simulink model "Copy_of_NDI"  (R2024b)
settings: Solver=ode4  StartTime=0  StopTime=100  FixedStep=fcs.Ts  RelTol=1e-3
PreLoadFcn:
  | FlightPhase = 'FallingLeaf';
  | % FlightPhase = 'InAir';
  | % FlightPhase = 'TVC_h10000V617alpha2';
  | run('PreLoadFcn.m')
values from neighbouring files (symbols this model uses):
  ControlAllocation = 1    [PreLoadFcn.m]    (also in RunThis_ChiaWei.m = 4; RunThis_LM.m = 4; RunThis_Shao.m; RunThis_james.m = 10)
  DUmax = IN_MAT(k+4,1:m)'    [LP_def.m]    (also in LP_lift.m; LP_sig.m; LP_thrust.m; PreLoadFcn.m = [Aactuator.right_aileron.RateLimitUpper Aactuator.left_ailer)
  DUmin = IN_MAT(k+5,1:m)'    [LP_def.m]    (also in LP_lift.m; LP_sig.m; LP_thrust.m; PreLoadFcn.m = [Aactuator.right_aileron.RateLimitLower Aactuator.left_ailer)
  g = [ 0  0  32.17 ]    [PreLoadFcn.m]
  hground = 0    [PreLoadFcn.m]
  m = m1-1    [CGIwrap.m]    (also in DAISY_CHAINING.m; DA_Allocation.m; LP_BasicSolution.m; LP_def.m)
  Mode_deflection_aileron = 1    [PreLoadFcn.m]    (also in RunThis_ChiaWei.m; RunThis_Shao.m = 0)
  Mode_deflection_elevator = 1    [PreLoadFcn.m]    (also in RunThis_ChiaWei.m; RunThis_Shao.m = 0)
  Mode_deflection_rudder = 1    [PreLoadFcn.m]    (also in RunThis_ChiaWei.m; RunThis_Shao.m = 0)
  Mode_deflection_TVC_y = 1    [PreLoadFcn.m]    (also in RunThis_ChiaWei.m; RunThis_Shao.m = 2)
  Mode_deflection_TVC_z = 1    [PreLoadFcn.m]    (also in RunThis_ChiaWei.m; RunThis_Shao.m = 0)
  N = IN_MAT(k+7:k+15,1:m)    [CGIwrap.m]    (also in DAISY_CHAINING.m; PreLoadFcn.m = [ 1      0     0.25; RunThis_ChiaWei.m = [ 1      0     0.25; RunThis_LM.m = [ 1      0     0.25)
  Ninv_2nozzle = inv(diag([  1/21.5  1/21.5  1/25  1/25  1/30  1/15  1/15  1/15  1/15 ]))    [PreLoadFcn.m]
  Ninv_no_nozzle = diag([    21.5    21.5    25    25    30    0     0     0     0  ])    [PreLoadFcn.m]
  state0 = [IC.npos IC.epos IC.alt IC.q0 IC.q1 IC.q2 IC.q3  IC.p IC.q IC.r IC.alpha IC.beta IC.mu IC.Vt IC.chi IC.gamma]    [PreLoadFcn.m]
  Umax_2nozzle = [Aactuator.right_aileron.AngleLimitUpper  Aactuator.left_aileron.AngleLimitUpper  Aactuator.right_elevator.AngleLimitUpper Aactuator.left_elevator.AngleLimitUpper  Aactuator.rudder.AngleLimitUpper                  Aactuator.TVC_ry.AngleLimitUpper    Aactuator.TVC_rz.AngleLimitUpper  Aactuator.TVC_ly.AngleLimitUpper    Aactuator.TVC_lz.AngleLimitUpper]    [PreLoadFcn.m]
  Umax_no_nozzle = [Aactuator.right_aileron.AngleLimitUpper  Aactuator.left_aileron.AngleLimitUpper  Aactuator.right_elevator.AngleLimitUpper Aactuator.left_elevator.AngleLimitUpper  Aactuator.rudder.AngleLimitUpper                    0 0 0 0]    [PreLoadFcn.m]
  Umin_2nozzle = [Aactuator.aileron.AngleLimitLower  Aactuator.aileron.AngleLimitLower  Aactuator.elevator.AngleLimitLower Aactuator.elevator.AngleLimitLower  Aactuator.rudder.AngleLimitLower                  Aactuator.TVC_ry.AngleLimitLower    Aactuator.TVC_rz.AngleLimitLower Aactuator.TVC_ly.AngleLimitLower    Aactuator.TVC_lz.AngleLimitLower]    [PreLoadFcn.m]
  Umin_no_nozzle = [Aactuator.right_aileron.AngleLimitLower  Aactuator.left_aileron.AngleLimitLower  Aactuator.right_elevator.AngleLimitLower Aactuator.left_elevator.AngleLimitLower  Aactuator.rudder.AngleLimitLower                    0 0 0 0]    [PreLoadFcn.m]
undefined symbols (not defined in the file or in its folder): Aactuator, ac, AeroCoeff, EngineTable, F, fcs, ft, IC, kg, LandingGear, Light, MIL, PIController, s, Sensor, sigbuilder_block, slug, sysID_DAQ, sysID_OBES, WMM2020
libraries: aerolibconvert2 x31, slpidlib x11, simulink x6, sharedutil x4, aerolibatmos2 x3, aerolibwind2 x3, aerolibbdyn x3, aerolibgravity2 x2, sharedtransform x1
(part 13 of 14)

== system Copy_of_NDI/F-16 Vehicle Systems Model/Vehicle/Aerodynamics/Aerofynamic Coefficients/CZT ==
  note: 氣動力表格僅提供到攻角到
      | 45度，超過45度後皆採用45
      | 度的氣動力係數
  note: ${\hat{Z} }_{\delta_e } =\frac{C_Z {\left(\alpha ,\beta ,\delta_e +0.1\right)}-C_Z {\left(\alpha ,\beta ,\delta_e -0.1\right)}}{0.2}$
  note: $\Delta C_{Z_{LEF} } =C_{Z_{LEF} } {\left(\alpha ,\beta \right)}-C_Z {\left(\alpha ,\beta ,\delta_e =0°\right)}$
  note: $C_{Z,T} =C_Z {\left(\alpha ,\beta ,\delta_e \right)}+\Delta C_{Z_{LEF} } ∙{\left(1-\frac{\delta_{LEF} }{25°}\right)}+\frac{q\overset{-}{c} }{2V_T }∙{\left[C_{Z_q } {\left(\alpha \right)}+\Delta C_{Z_{q_{LEF} } } {\left(\alpha \right)}∙{\left(1-\frac{\delta_{LEF} }{25°}\right)}\right]}+\ \Delta C_{Z_{SB} } {\left(\alpha \right)}∙{\left(\frac{\delta_{SB} }{60°}\right)}+C_{Z_{\delta ra} } \delta_{ra} +C_{Z_{\delta la} } \delta_{la}$
  note: $C_{Z_{\delta ra} } =C_{Z_{\delta la} } =\frac{{\hat{Z} }_{\delta_e } }{2}∙0.4$
  note: 體軸 z 方向之氣動力係數 (total z-axis force coefficient)：
  note: ${\hat{Z} }_{\delta_e } =\frac{C_Z {\left(\alpha ,\beta ,\delta_e +0.1\right)}-C_Z {\left(\alpha ,\beta ,\delta_e -0.1\right)}}{0.2}$
  note: $C_{Z_{\delta ra} } =C_{Z_{\delta la} } =\frac{{\hat{Z} }_{\delta_e } }{2}∙0.4$
  alpha (deg) : Inport
  beta (deg) : Inport  Port=2
  right elevator (deg) : Inport  Port=3
  left elevator (deg) : Inport  Port=4
  dlef : Inport  Port=5
  qc_2v : Inport  Port=6
  sb : Inport  Port=7
  right aileron : Inport  Port=8
  left aileron : Inport  Port=9
  Add : Sum  Inputs=+-
  Add1 : Sum  Inputs=+++++
  Add{2..4,7} (4 alike) : Sum
  Add5 : Sum  Inputs=+-
  Add6 : Sum  Inputs=+-
  CZ : Interpolation_n-D  NumberOfTableDimensions=3  Table=AeroCoeff.CZ
      settings: InputPortMap=u0,u1,u2,u3,u4,u5
  CZ1 : Interpolation_n-D  NumberOfTableDimensions=3  Table=AeroCoeff.CZ
      settings: InputPortMap=u0,u1,u2,u3,u4,u5
  CZ2 : Interpolation_n-D  NumberOfTableDimensions=3  Table=AeroCoeff.CZ
      settings: InputPortMap=u0,u1,u2,u3,u4,u5
  CZ_elevator0 : Interpolation_n-D  Table=AeroCoeff.CZ_elevator0
  CZ_lef : Interpolation_n-D  Table=AeroCoeff.CZ_lef
  CZ_q : Interpolation_n-D  NumberOfTableDimensions=1  Table=AeroCoeff.CZ_q
      settings: InputPortMap=u0,u1
  Constant : Constant  Value=0.1
  Constant1 : Constant  Value=0.1
  Constant2 : Constant  Value=0.2
  Divide : Product  Inputs=*/
  Gain : Gain  Gain=20
  Gain2 : Gain  Gain=(1/2)*0.4
  Gain3 : Gain  Gain=20
  Gain4 : Gain  Gain=1/2
  Product{,1..5} (6 alike) : Product
  alpha Prelookup : PreLookup  BreakpointsData=AeroCoeff.alpha_prelookup  IndexSearchMethod=Linear search  BeginIndexSearchUsingPreviousIndexResult=on  DiagnosticForOutOfRangeInput=Warning
  beta Prelookup : PreLookup  BreakpointsData=AeroCoeff.beta_prelookup  IndexSearchMethod=Linear search  BeginIndexSearchUsingPreviousIndexResult=on  DiagnosticForOutOfRangeInput=Warning
  dCZ_q_lef : Interpolation_n-D  NumberOfTableDimensions=1  Table=AeroCoeff.dCZ_q_lef
      settings: InputPortMap=u0,u1
  dCZ_sb : Interpolation_n-D  NumberOfTableDimensions=1  Table=AeroCoeff.dCZ_sb
      settings: InputPortMap=u0,u1
  elevator Prelookup : PreLookup  BreakpointsData=AeroCoeff.elevator_prelookup2  IndexSearchMethod=Linear search  BeginIndexSearchUsingPreviousIndexResult=on  DiagnosticForOutOfRangeInput=Warning
  elevator Prelookup1 : PreLookup  BreakpointsData=AeroCoeff.elevator_prelookup2  IndexSearchMethod=Linear search  BeginIndexSearchUsingPreviousIndexResult=on  DiagnosticForOutOfRangeInput=Warning
  elevator Prelookup2 : PreLookup  BreakpointsData=AeroCoeff.elevator_prelookup2  IndexSearchMethod=Linear search  BeginIndexSearchUsingPreviousIndexResult=on  DiagnosticForOutOfRangeInput=Warning
  Cz_tot : Outport  VectorParamsAs1DForOutWhenUnconnected=off
  wires:
  Product2/1 -> Add1/3
  alpha Prelookup/2 -> dCZ_q_lef/2, dCZ_sb/2, CZ2/2, CZ1/2, CZ_q/2, CZ_elevator0/2, CZ_lef/2, CZ/2
  Add1/1 -> Cz_tot/1
  elevator Prelookup/1 -> CZ/5
  CZ_q/1 -> Add2/1
  beta Prelookup/2 -> CZ/4, CZ_lef/4, CZ_elevator0/4, CZ2/4, CZ1/4
  CZ_lef/1 -> Add/1
  dCZ_q_lef/1 -> Product1/1
  Product1/1 -> Add2/2
  Add2/1 -> Product2/1
  CZ_elevator0/1 -> Add/2
  Add/1 -> Product/1
  dlef/1 -> Product1/2, Product/2
  Product/1 -> Add1/2
  CZ/1 -> Add1/1
  beta Prelookup/1 -> CZ/3, CZ_elevator0/3, CZ2/3, CZ1/3, CZ_lef/3
  alpha Prelookup/1 -> dCZ_q_lef/1, CZ1/1, CZ2/1, dCZ_sb/1, CZ_q/1, CZ_elevator0/1, CZ_lef/1, CZ/1
  alpha (deg)/1 -> alpha Prelookup/1
  elevator Prelookup/2 -> CZ/6
  qc_2v/1 -> Product2/2
  beta (deg)/1 -> beta Prelookup/1
  sb/1 -> Product3/2
  dCZ_sb/1 -> Product3/1
  Product3/1 -> Add1/4
  Constant1/1 -> Add5/2
  CZ2/1 -> Add6/2
  Constant/1 -> Add4/2
  Add5/1 -> elevator Prelookup2/1
  Product5/1 -> Add7/2
  Add4/1 -> elevator Prelookup1/1
  left aileron/1 -> Gain3/1
  Divide/1 -> Gain2/1
  right aileron/1 -> Gain/1
  Add6/1 -> Divide/1
  Gain2/1 -> Product5/1, Product4/1
  CZ1/1 -> Add6/1
  Product4/1 -> Add7/1
  Add3/1 -> Gain4/1
  right elevator (deg)/1 -> Add3/1
  left elevator (deg)/1 -> Add3/2
  elevator Prelookup1/1 -> CZ1/5
  elevator Prelookup1/2 -> CZ1/6
  elevator Prelookup2/1 -> CZ2/5
  elevator Prelookup2/2 -> CZ2/6
  Constant2/1 -> Divide/2
  Add7/1 -> Add1/5
  Gain/1 -> Product4/2
  Gain3/1 -> Product5/2
  Gain4/1 -> elevator Prelookup/1, Add5/1, Add4/1

== system Copy_of_NDI/F-16 Vehicle Systems Model/Vehicle/Aerodynamics/Aerofynamic Coefficients/ClT ==
  note: $\Delta C_{l_{\delta_a } }$
  note: $\Delta C_{l_{{\delta_a }_{LEF} } } =C_{l_{{\delta_a =20°}_{LEF} } } {\left(\alpha ,\beta \right)}-C_{l_{LEF} } {\left(\alpha ,\beta \right)}-\Delta C_{l_{\delta_a } }$
  note: $\Delta C_{l_{\delta_r } } =C_{l_{\delta_r =30°} } {\left(\alpha ,\beta \right)}-C_l {\left(\alpha ,\beta ,\delta_e =0°\right)}$
  note: $\Delta C_{l_{\delta_a } } =C_{l_{\delta_a =20°} } {\left(\alpha ,\beta \right)}-C_l {\left(\alpha ,\beta ,\delta_e =0°\right)}$
  note: $\Delta C_{l_{LEF} } =C_{l_{LEF} } {\left(\alpha ,\beta \right)}-C_l {\left(\alpha ,\beta ,\delta_e =0°\right)}$
  note: 側滾氣動力矩係數 (total rolling moment coefficient)：
  note: 氣動力表格僅提供到攻角到
      | 45度，超過45度後皆採用45
      | 度的氣動力係數
  note: 氣動力表格僅提供到攻角到
      | 45度，超過45度後皆採用45
      | 度的氣動力係數
  note: $C_{l,T} \ \ \ =\ \ \ C_l {\left(\alpha ,\beta ,\delta_e \right)}+\Delta C_{l_{LEF} } ∙{\left(1-\frac{\delta_{LEF} }{25°}\right)}+\frac{pb}{2V_T }∙{\left[C_{l_p } {\left(\alpha \right)}+\Delta C_{l_{p_{LEF} } } {\left(\alpha \right)}∙{\left(1-\frac{\delta_{LEF} }{25°}\right)}\right]}+\frac{rb}{2V_T }∙{\left[C_{l_r } {\left(\alpha \right)}+\Delta C_{l_{r_{LEF} } } {\left(\alpha \right)}∙{\left(1-\frac{\delta_{LEF} }{25°}\right)}\right]}+\Delta C_{l_{\beta } } {\left(\alpha \right)}∙\beta +\Delta C_{l_{\delta_r } } ∙{\left(\frac{\delta_r }{30°}\right)}+\frac{{\left[\Delta C_{l_{\delta_a } } +\Delta C_{l_{{\delta_a }_{LEF} } } ∙{\left(1-\frac{\delta_{LEF} }{25°}\right)}\right]}}{2}∙{\left(\frac{\delta_{ra} }{20°}\right)}-\frac{{\left[\Delta C_{l_{\delta_a } } +\Delta C_{l_{{\delta_a }_{LEF} } } ∙{\left(1-\frac{\delta_{LEF} }{25°}\right)}\right]}}{2}∙{\left(\frac{\delta_{la} }{20°}\right)}+C_{l_{\delta re} } ∙{\left(\frac{\delta_{re} }{25°}\right)}-C_{l_{\delta le} } ∙{\left(\frac{\delta_{le} }{25°}\right)}$
  note: $C_{l_{\delta re} } =C_{l_{\delta le} } =\frac{\Delta C_{l_{\delta_a } } }{2}∙0.56$
  note: $\Delta C_{l_{\delta_a } }$
  note: $C_{l_{\delta re} } =C_{l_{\delta le} } =\frac{\Delta C_{l_{\delta_a } } }{2}∙0.56$
  alpha (deg) : Inport
  beta (deg) : Inport  Port=2
  drud : Inport  Port=3
  dlef : Inport  Port=4
  right aileron : Inport  Port=5
  left aileron : Inport  Port=6
  rb_2v : Inport  Port=7
  pb_2v : Inport  Port=8
  right elevator (deg) : Inport  Port=9
  left elevator (deg) : Inport  Port=10
  Add : Sum  Inputs=+-
  Add1 : Sum  Inputs=+-
  Angle Conversion : aerolibconvert2/Angle Conversion  IU=deg  OU=rad
  Cl : Interpolation_n-D  NumberOfTableDimensions=3  Table=AeroCoeff.Cl
      settings: InputPortMap=u0,u1,u2,u3,u4,u5
  Cl_delta_ail : Interpolation_n-D  Table=AeroCoeff.Cl_delta_ail  InternalRulePriority=Speed
  Cl_delta_ail_lef : Interpolation_n-D  Table=AeroCoeff.Cl_delta_ail_lef  InternalRulePriority=Speed
  Cl_delta_r : Interpolation_n-D  Table=AeroCoeff.Cl_delta_r  InternalRulePriority=Speed
  Cl_elevator0 : Interpolation_n-D  Table=AeroCoeff.Cl_elevator0
  Cl_lef : Interpolation_n-D  Table=AeroCoeff.Cl_lef  InternalRulePriority=Speed
  Cl_p : Interpolation_n-D  NumberOfTableDimensions=1  Table=AeroCoeff.Cl_p  InternalRulePriority=Speed
      settings: InputPortMap=u0,u1
  Cl_r : Interpolation_n-D  NumberOfTableDimensions=1  Table=AeroCoeff.Cl_r  InternalRulePriority=Speed
      settings: InputPortMap=u0,u1
  Gain : Gain  Gain=1/2
  Gain1 : Gain  Gain=1/25
  Gain2 : Gain  Gain=(1/2)*0.56
  Product{,1..9} (10 alike) : Product
  Subtract : Sum  Inputs=+-
  Subtract1 : Sum  Inputs=+-
  Subtract2 : Sum  Inputs=+--
  Subtract3 : Sum  Inputs=+-
  Subtract4 : Sum  Inputs=++++++++
  Subtract5 : Sum
  Subtract6 : Sum
  Subtract7 : Sum
  alpha Prelookup : PreLookup  BreakpointsData=AeroCoeff.alpha_prelookup  IndexSearchMethod=Linear search  BeginIndexSearchUsingPreviousIndexResult=on  DiagnosticForOutOfRangeInput=Warning
  beta Prelookup : PreLookup  BreakpointsData=AeroCoeff.beta_prelookup  IndexSearchMethod=Linear search  BeginIndexSearchUsingPreviousIndexResult=on  DiagnosticForOutOfRangeInput=Warning
  dCl_beta : Interpolation_n-D  NumberOfTableDimensions=1  Table=AeroCoeff.dCl_beta  InternalRulePriority=Speed
      settings: InputPortMap=u0,u1
  dCl_p_lef : Interpolation_n-D  NumberOfTableDimensions=1  Table=AeroCoeff.dCl_p_lef  InternalRulePriority=Speed
      settings: InputPortMap=u0,u1
  dCl_r_lef : Interpolation_n-D  NumberOfTableDimensions=1  Table=AeroCoeff.dCl_r_lef  InternalRulePriority=Speed
      settings: InputPortMap=u0,u1
  elevator Prelookup : PreLookup  BreakpointsData=AeroCoeff.elevator_prelookup1  IndexSearchMethod=Linear search  BeginIndexSearchUsingPreviousIndexResult=on  DiagnosticForOutOfRangeInput=Warning
  Cl_tot : Outport  VectorParamsAs1DForOutWhenUnconnected=off
  wires:
  Cl_elevator0/1 -> Subtract3/2, Subtract1/2, Subtract/2
  beta Prelookup/1 -> Cl/3, Cl_lef/3, Cl_elevator0/3, Cl_delta_r/3, Cl_delta_ail_lef/3, Cl_delta_ail/3
  Cl_delta_r/1 -> Subtract3/1
  Cl_lef/1 -> Subtract2/3, Subtract/1
  Subtract/1 -> Product/1
  Product6/1 -> Subtract7/2
  alpha Prelookup/1 -> Cl/1, Cl_lef/1, dCl_r_lef/1, dCl_p_lef/1, dCl_beta/1, Cl_p/1, Cl_r/1, Cl_delta_r/1, Cl_delta_ail_lef/1, Cl_delta_ail/1, Cl_elevator0/1
  Product2/1 -> Subtract4/3
  Cl_p/1 -> Subtract7/1
  beta (deg)/1 -> beta Prelookup/1, Angle Conversion/1
  Subtract2/1 -> Product1/1
  alpha Prelookup/2 -> Cl/2, Cl_lef/2, Cl_r/2, dCl_r_lef/2, dCl_p_lef/2, dCl_beta/2, Cl_p/2, Cl_delta_r/2, Cl_delta_ail_lef/2, Cl_delta_ail/2, Cl_elevator0/2
  alpha (deg)/1 -> alpha Prelookup/1
  Product/1 -> Subtract4/2
  Subtract6/1 -> Product5/2
  rb_2v/1 -> Product5/1
  Cl_delta_ail/1 -> Subtract1/1
  Subtract5/1 -> Product2/1
  drud/1 -> Product3/2
  elevator Prelookup/1 -> Cl/5
  Product7/1 -> Subtract4/6
  Subtract7/1 -> Product7/1
  Product5/1 -> Subtract4/5
  dCl_r_lef/1 -> Product4/1
  Subtract3/1 -> Product3/1
  Subtract1/1 -> Subtract2/2, Subtract5/1, [delta_Cl_delta_ail]
  dlef/1 -> Product6/1, Product4/2, Product/2, Product1/2
  Product3/1 -> Subtract4/4
  Cl_delta_ail_lef/1 -> Subtract2/1
  beta Prelookup/2 -> Cl/4, Cl_lef/4, Cl_elevator0/4, Cl_delta_ail/4, Cl_delta_r/4, Cl_delta_ail_lef/4
  Product4/1 -> Subtract6/2
  dCl_beta/1 -> Product8/1
  Product1/1 -> Subtract5/2
  dCl_p_lef/1 -> Product6/2
  Product8/1 -> Subtract4/7
  Cl_r/1 -> Subtract6/1
  elevator Prelookup/2 -> Cl/6
  Cl/1 -> Subtract4/1
  Subtract4/1 -> Cl_tot/1
  pb_2v/1 -> Product7/2
  right aileron/1 -> Add/1
  left aileron/1 -> Add/2
  Add/1 -> Gain/1
  Gain/1 -> Product2/2
  right elevator (deg)/1 -> Add1/1
  left elevator (deg)/1 -> Add1/2
  Add1/1 -> Gain1/1, elevator Prelookup/1
  Gain1/1 -> Product9/2
  [delta_Cl_delta_ail] -> Gain2/1
  Gain2/1 -> Product9/1
  Product9/1 -> Subtract4/8
  Angle Conversion/1 -> Product8/2

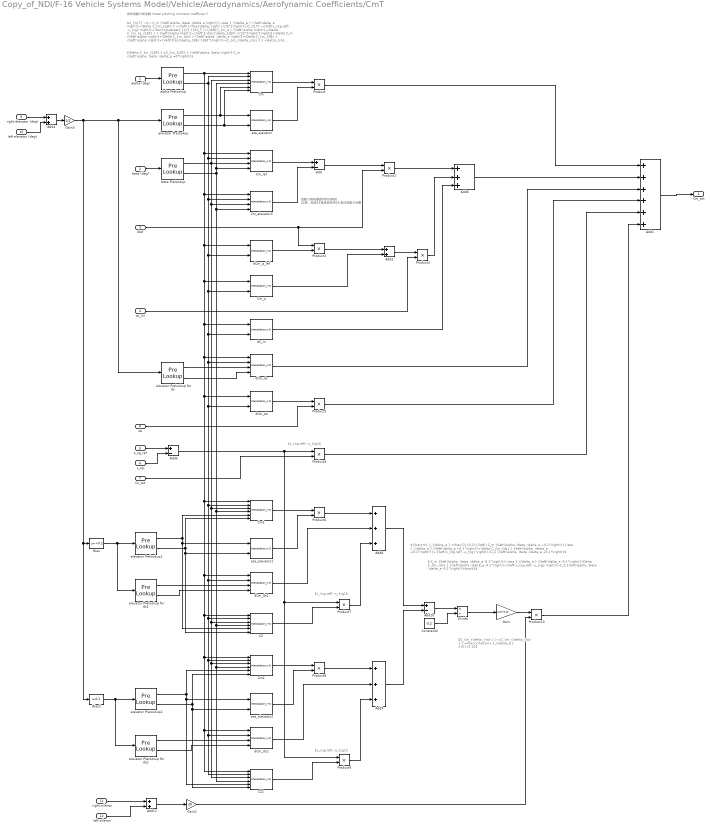
== system Copy_of_NDI/F-16 Vehicle Systems Model/Vehicle/Aerodynamics/Aerofynamic Coefficients/CmT ==
  note: 氣動力表格僅提供到攻角到
      | 45度，超過45度後皆採用45
      | 度的氣動力係數
  note: $x_{cg,ref} -x_{cg}$
  note: 俯仰氣動力矩係數 (total pitching moment coefficient)：
  note: $\Delta C_{m_{LEF} } =C_{m_{LEF} } {\left(\alpha ,\beta \right)}-C_m {\left(\alpha ,\beta ,\delta_e =0°\right)}$
  note: $C_{m,T} \ =\ \ C_m {\left(\alpha ,\beta ,\delta_e \right)}{∙\eta }_{\delta_e } {\left(\delta_e \right)}+\Delta C_{m_{LEF} } ∙{\left(1-\frac{\delta_{LEF} }{25°}\right)}+C_{Z,T} ∙{\left(x_{cg,ref} -x_{cg} \right)}+\frac{q\overset{-}{c} }{2V_T }∙{\left[C_{m_q } {\left(\alpha \right)}+\Delta C_{m_{q_{LEF} } } {\left(\alpha \right)}∙{\left(1-\frac{\delta_{LEF} }{25°}\right)}\right]}+\Delta C_m {\left(\alpha \right)}+\Delta C_{m_{ds} } {\left(\alpha ,\delta_e \right)}+\Delta C_{m_{SB} } {\left(\alpha \right)}∙{\left(\frac{\delta_{SB} }{60°}\right)}+C_{m_{\delta_{ra} } } ∙\delta_{ra} +C_{m_{\delta_{la} } } ∙\delta_{la}$
  note: $-C_m {\left(\alpha ,\beta ,\delta_e -0.1°\right)}{∙\eta }_{\delta_e } {\left(\delta_e -0.1°\right)}-\Delta C_{m_{ds} } {\left(\alpha ,\delta_e -0.1°\right)}-{\left(x_{cg,ref} -x_{cg} \right)}∙C_Z {\left(\alpha ,\beta ,\delta_e -0.1°\right)}\rbrack}$
  note: ${\hat{m} }_{\delta_e } =\frac{1}{0.2}{\left[\ C_m {\left(\alpha ,\beta ,\delta_e +0.1°\right)}{∙\eta }_{\delta_e } {\left(\delta_e +0.1°\right)}+\Delta C_{m_{ds} } {\left(\alpha ,\delta_e +0.1°\right)}}+{\left(x_{cg,ref} -x_{cg} \right)}∙C_Z {\left(\alpha ,\beta ,\delta_e +0.1°\right)}$
  note: $x_{cg,ref} -x_{cg}$
  note: $x_{cg,ref} -x_{cg}$
  note: $C_{m_{\delta_{ra} } } =C_{m_{\delta_{la} } } =\frac{{\hat{m} }_{\delta_e } }{2}∙0.12$
  alpha (deg) : Inport
  beta (deg) : Inport  Port=2
  dlef : Inport  Port=3
  qc_2v : Inport  Port=4
  x_cg_ref : Inport  Port=5
  x_cg : Inport  Port=6
  Cz_tot : Inport  Port=7
  sb : Inport  Port=8
  right elevator (deg) : Inport  Port=9
  left elevator (deg) : Inport  Port=10
  right aileron : Inport  Port=11
  left aileron : Inport  Port=12
  Add : Sum  Inputs=+-
  Add1 : Sum  Inputs=++++++
  Add10 : Sum  Inputs=+-
  Add11 : Sum
  Add2 : Sum
  Add3 : Sum  Inputs=+-
  Add4 : Sum
  Add6 : Sum  Inputs=+++
  Add8 : Sum  Inputs=+++
  Add9 : Sum  Inputs=+++
  Bias : Bias  Bias=+0.1  SaturateOnIntegerOverflow=off
  Bias1 : Bias  Bias=-0.1  SaturateOnIntegerOverflow=off
  CZ : Interpolation_n-D  NumberOfTableDimensions=3  Table=AeroCoeff.CZ
      settings: InputPortMap=u0,u1,u2,u3,u4,u5
  CZ1 : Interpolation_n-D  NumberOfTableDimensions=3  Table=AeroCoeff.CZ
      settings: InputPortMap=u0,u1,u2,u3,u4,u5
  Cm : Interpolation_n-D  NumberOfTableDimensions=3  Table=AeroCoeff.Cm
      settings: InputPortMap=u0,u1,u2,u3,u4,u5
  Cm1 : Interpolation_n-D  NumberOfTableDimensions=3  Table=AeroCoeff.Cm
      settings: InputPortMap=u0,u1,u2,u3,u4,u5
  Cm2 : Interpolation_n-D  NumberOfTableDimensions=3  Table=AeroCoeff.Cm
      settings: InputPortMap=u0,u1,u2,u3,u4,u5
  Cm_elevator0 : Interpolation_n-D  Table=AeroCoeff.Cm_elevator0
  Cm_lef : Interpolation_n-D  Table=AeroCoeff.Cm_lef
  Cm_q : Interpolation_n-D  NumberOfTableDimensions=1  Table=AeroCoeff.Cm_q
      settings: InputPortMap=u0,u1
  Constant2 : Constant  Value=0.2
  Divide : Product  Inputs=*/
  Gain : Gain  Gain=(1/2)*0.12
  Gain2 : Gain  Gain=20
  Gain3 : Gain  Gain=1/2
  Product{,1..10} (11 alike) : Product
  alpha Prelookup : PreLookup  BreakpointsData=AeroCoeff.alpha_prelookup  IndexSearchMethod=Linear search  BeginIndexSearchUsingPreviousIndexResult=on  DiagnosticForOutOfRangeInput=Warning
  beta Prelookup : PreLookup  BreakpointsData=AeroCoeff.beta_prelookup  IndexSearchMethod=Linear search  BeginIndexSearchUsingPreviousIndexResult=on  DiagnosticForOutOfRangeInput=Warning
  dC_m : Interpolation_n-D  NumberOfTableDimensions=1  Table=AeroCoeff.dC_m
      settings: InputPortMap=u0,u1
  dCm_ds : Interpolation_n-D  Table=AeroCoeff.dCm_ds
  dCm_ds1 : Interpolation_n-D  Table=AeroCoeff.dCm_ds
  dCm_ds2 : Interpolation_n-D  Table=AeroCoeff.dCm_ds
  dCm_q_lef : Interpolation_n-D  NumberOfTableDimensions=1  Table=AeroCoeff.dCm_q_lef
      settings: InputPortMap=u0,u1
  dCm_sb : Interpolation_n-D  NumberOfTableDimensions=1  Table=AeroCoeff.dCm_sb
      settings: InputPortMap=u0,u1
  elevator Prelookup : PreLookup  BreakpointsData=AeroCoeff.elevator_prelookup2  IndexSearchMethod=Linear search  BeginIndexSearchUsingPreviousIndexResult=on  DiagnosticForOutOfRangeInput=Warning
  elevator Prelookup for ds : PreLookup  BreakpointsData=AeroCoeff.elevator_prelookup3  IndexSearchMethod=Linear search  BeginIndexSearchUsingPreviousIndexResult=on  DiagnosticForOutOfRangeInput=Warning
  elevator Prelookup for ds1 : PreLookup  BreakpointsData=AeroCoeff.elevator_prelookup3  IndexSearchMethod=Linear search  BeginIndexSearchUsingPreviousIndexResult=on  DiagnosticForOutOfRangeInput=Warning
  elevator Prelookup for ds2 : PreLookup  BreakpointsData=AeroCoeff.elevator_prelookup3  IndexSearchMethod=Linear search  BeginIndexSearchUsingPreviousIndexResult=on  DiagnosticForOutOfRangeInput=Warning
  elevator Prelookup1 : PreLookup  BreakpointsData=AeroCoeff.elevator_prelookup2  IndexSearchMethod=Linear search  BeginIndexSearchUsingPreviousIndexResult=on  DiagnosticForOutOfRangeInput=Warning
  elevator Prelookup2 : PreLookup  BreakpointsData=AeroCoeff.elevator_prelookup2  IndexSearchMethod=Linear search  BeginIndexSearchUsingPreviousIndexResult=on  DiagnosticForOutOfRangeInput=Warning
  eta_elevator : Interpolation_n-D  NumberOfTableDimensions=1  Table=AeroCoeff.eta_elevator
      settings: InputPortMap=u0,u1
  eta_elevator1 : Interpolation_n-D  NumberOfTableDimensions=1  Table=AeroCoeff.eta_elevator
      settings: InputPortMap=u0,u1
  eta_elevator2 : Interpolation_n-D  NumberOfTableDimensions=1  Table=AeroCoeff.eta_elevator
      settings: InputPortMap=u0,u1
  Cm_tot : Outport  VectorParamsAs1DForOutWhenUnconnected=off
  wires:
  Cm/1 -> Product/1
  Cm_lef/1 -> Add/1
  Add3/1 -> Product4/1, Product7/1, Product9/1
  alpha Prelookup/1 -> Cm1/1, dCm_ds2/1, CZ1/1, Cm2/1, CZ/1, dCm_ds1/1, dCm_sb/1, dCm_ds/1, dC_m/1, Cm_q/1, dCm_q_lef/1, Cm_elevator0/1, Cm_lef/1, Cm/1
  Cm_elevator0/1 -> Add/2
  elevator Prelookup/1 -> eta_elevator/1, Cm/5
  dC_m/1 -> Add6/3
  alpha Prelookup/2 -> Cm1/2, dCm_ds1/2, Cm2/2, dCm_ds2/2, CZ1/2, CZ/2, dCm_sb/2, dCm_ds/2, dC_m/2, Cm_q/2, dCm_q_lef/2, Cm_elevator0/2, Cm_lef/2, Cm/2
  dlef/1 -> Product2/1, Product1/2
  elevator Prelookup/2 -> eta_elevator/2, Cm/6
  Add4/1 -> Gain3/1
  eta_elevator/1 -> Product/2
  beta Prelookup/2 -> Cm/4, Cm_lef/4, Cm1/4, CZ/4, Cm2/4, CZ1/4, Cm_elevator0/4
  Product2/1 -> Add2/1
  Cm_q/1 -> Add2/2
  beta Prelookup/1 -> Cm/3, Cm1/3, CZ/3, Cm2/3, CZ1/3, Cm_elevator0/3, Cm_lef/3
  dCm_q_lef/1 -> Product2/2
  Add2/1 -> Product3/1
  Add/1 -> Product1/1
  qc_2v/1 -> Product3/2
  alpha (deg)/1 -> alpha Prelookup/1
  Product4/1 -> Add1/5
  beta (deg)/1 -> beta Prelookup/1
  x_cg/1 -> Add3/2
  Add1/1 -> Cm_tot/1
  Cz_tot/1 -> Product4/2
  x_cg_ref/1 -> Add3/1
  sb/1 -> Product5/2
  dCm_sb/1 -> Product5/1
  Product5/1 -> Add1/4
  elevator Prelookup for ds/1 -> dCm_ds/3
  elevator Prelookup for ds/2 -> dCm_ds/4
  dCm_ds/1 -> Add1/3
  Product1/1 -> Add6/1
  Product3/1 -> Add6/2
  Add6/1 -> Add1/2
  Product/1 -> Add1/1
  right elevator (deg)/1 -> Add4/1
  left elevator (deg)/1 -> Add4/2
  eta_elevator1/1 -> Product6/2
  Cm1/1 -> Product6/1
  elevator Prelookup1/1 -> Cm1/5, eta_elevator1/1, CZ/5
  elevator Prelookup1/2 -> Cm1/6, eta_elevator1/2, CZ/6
  Bias/1 -> elevator Prelookup1/1, elevator Prelookup for ds1/1
  elevator Prelookup for ds1/1 -> dCm_ds1/3
  elevator Prelookup for ds1/2 -> dCm_ds1/4
  Product6/1 -> Add8/1
  dCm_ds1/1 -> Add8/2
  CZ/1 -> Product7/2
  Product7/1 -> Add8/3
  Bias1/1 -> elevator Prelookup2/1, elevator Prelookup for ds2/1
  elevator Prelookup2/1 -> eta_elevator2/1, CZ1/5, Cm2/5
  elevator Prelookup2/2 -> eta_elevator2/2, CZ1/6, Cm2/6
  elevator Prelookup for ds2/1 -> dCm_ds2/3
  elevator Prelookup for ds2/2 -> dCm_ds2/4
  Cm2/1 -> Product8/1
  eta_elevator2/1 -> Product8/2
  Product8/1 -> Add9/1
  dCm_ds2/1 -> Add9/2
  CZ1/1 -> Product9/2
  Product9/1 -> Add9/3
  Add8/1 -> Add10/1
  Add9/1 -> Add10/2
  Add10/1 -> Divide/1
  Constant2/1 -> Divide/2
  Divide/1 -> Gain/1
  Gain/1 -> Product10/1
  right aileron/1 -> Add11/1
  left aileron/1 -> Add11/2
  Add11/1 -> Gain2/1
  Product10/1 -> Add1/6
  Gain2/1 -> Product10/2
  Gain3/1 -> elevator Prelookup/1, elevator Prelookup for ds/1, Bias1/1, Bias/1

== system Copy_of_NDI/F-16 Vehicle Systems Model/Vehicle/Aerodynamics/Aerofynamic Coefficients/CnT ==
  note: $\Delta C_{n_{\delta_a } }$
  note: 氣動力表格僅提供到攻角到
      | 45度，超過45度後皆採用45
      | 度的氣動力係數
  note: 氣動力表格僅提供到攻角到
      | 45度，超過45度後皆採用45
      | 度的氣動力係數
  note: $C_n {\left(\alpha ,\beta ,\delta_e =0°\right)}$
  note: $C_{n_{\delta_r =30°} } {\left(\alpha ,\beta \right)}$
  note: $\Delta C_{n_{\delta_r } } =C_{n_{\delta_r =30°} } {\left(\alpha ,\beta \right)}-C_n {\left(\alpha ,\beta ,\delta_e =0°\right)}$
  note: $x_{cg,ref} -x_{cg}$
  note: $\frac{\bar{c} }{b}$
  note: $\Delta C_{n_{\delta_a } } =C_{n_{\delta_a =20°} } {\left(\alpha ,\beta \right)}-C_n {\left(\alpha ,\beta ,\delta_e =0°\right)}$
  note: $\Delta C_{n_{\delta_r } } =C_{n_{\delta_r =30°} } {\left(\alpha ,\beta \right)}-C_n {\left(\alpha ,\beta ,\delta_e =0°\right)}$
  note: $\ C_{n,T} \ \ =\ \ \ \ C_n {\left(\alpha ,\beta ,\delta_e \right)}+\Delta C_{n_{LEF} } ∙{\left(1-\frac{\delta_{LEF} }{25°}\right)}-C_{Y,T} ∙{\left(x_{cg,ref} -x_{cg} \right)}∙\frac{\overset{-}{c} }{b}+\frac{pb}{2V_T }∙{\left[C_{n_p } {\left(\alpha \right)}+\Delta C_{n_{p_{LEF} } } {\left(\alpha \right)}∙{\left(1-\frac{\delta_{LEF} }{25°}\right)}\right]}+\frac{rb}{2V_T }∙{\left[C_{n_r } {\left(\alpha \right)}+\Delta C_{n_{r_{LEF} } } {\left(\alpha \right)}∙{\left(1-\frac{\delta_{LEF} }{25°}\right)}\right]}+\Delta C_{n_{\beta } } {\left(\alpha \right)}∙\beta +\Delta C_{n_{\delta_r } } ∙{\left(\frac{\delta_r }{30°}\right)}+\frac{{\left[\Delta C_{n_{\delta_a } } +\Delta C_{n_{{\delta_a }_{LEF} } } ∙{\left(1-\frac{\delta_{LEF} }{25°}\right)}\right]}}{2}∙{\left(\frac{\delta_{ra} }{20°}\right)}-\frac{{\left[\Delta C_{n_{\delta_a } } +\Delta C_{n_{{\delta_a }_{LEF} } } ∙{\left(1-\frac{\delta_{LEF} }{25°}\right)}\right]}}{2}∙{\left(\frac{\delta_{la} }{20°}\right)}+C_{n_{\delta_{re} } } ∙{\left(\frac{\delta_{re} }{30°}\right)}-C_{n_{\delta_{le} } } ∙{\left(\frac{\delta_{le} }{30°}\right)}$
  note: $\Delta C_{n_{LEF} } =C_{n_{LEF} } {\left(\alpha ,\beta \right)}-C_n {\left(\alpha ,\beta ,\delta_e =0°\right)}$
  note: 偏航氣動力矩係數 (total yawing moment coefficient)：
  note: $\Delta C_{n_{{\delta_a }_{LEF} } } =C_{n_{{\delta_a =20°}_{LEF} } } {\left(\alpha ,\beta \right)}-C_{n_{LEF} } {\left(\alpha ,\beta \right)}-\Delta C_{n_{\delta_a } }$
  note: $\Delta C_{n_{\delta_a } }$
  note: $C_{n_{\delta_{re} } } =C_{n_{\delta_{le} } } =\frac{\Delta C_{n_{\delta_a } } }{2}∙0.26$
  alpha (deg) : Inport
  beta (deg) : Inport  Port=2
  right aileron : Inport  Port=3
  left aileron : Inport  Port=4
  "right elevator (deg) " : Inport  Port=5
  left elevator (deg) : Inport  Port=6
  drud : Inport  Port=7
  dlef : Inport  Port=8
  rb_2v : Inport  Port=9
  pb_2v : Inport  Port=10
  x_cg_ref : Inport  Port=11
  x_cg : Inport  Port=12
  cbar : Inport  Port=13
  b : Inport  Port=14
  Cy_tot : Inport  Port=15
  Add{,1,3,8..9,11} (6 alike) : Sum  Inputs=+-
  Add{5..7,10} (4 alike) : Sum
  Add2 : Sum  Inputs=--+
  Add4 : Sum  Inputs=++++++++-
  Angle Conversion : aerolibconvert2/Angle Conversion  IU=deg  OU=rad
  Cn : Interpolation_n-D  NumberOfTableDimensions=3  Table=AeroCoeff.Cn
      settings: InputPortMap=u0,u1,u2,u3,u4,u5
  Cn_delta_ail : Interpolation_n-D  Table=AeroCoeff.Cn_delta_ail
  Cn_delta_ail_lef : Interpolation_n-D  Table=AeroCoeff.Cn_delta_ail_lef
  Cn_delta_r : Interpolation_n-D  Table=AeroCoeff.Cn_delta_r
  Cn_elevator0 : Interpolation_n-D  Table=AeroCoeff.Cn_elevator0
  Cn_lef : Interpolation_n-D  Table=AeroCoeff.Cn_lef
  Cn_p : Interpolation_n-D  NumberOfTableDimensions=1  Table=AeroCoeff.Cn_p
      settings: InputPortMap=u0,u1
  Cn_r : Interpolation_n-D  NumberOfTableDimensions=1  Table=AeroCoeff.Cn_r
      settings: InputPortMap=u0,u1
  Divide : Product  Inputs=*/
  Gain : Gain  Gain=1/2
  Gain1 : Gain  Gain=1/25
  Gain2 : Gain  Gain=(1/2)*0.26
  Gain4 : Gain  Gain=1/2
  Product{,1..9} (10 alike) : Product
  Product10 : Product  Inputs=3
  alpha Prelookup : PreLookup  BreakpointsData=AeroCoeff.alpha_prelookup  IndexSearchMethod=Linear search  BeginIndexSearchUsingPreviousIndexResult=on  DiagnosticForOutOfRangeInput=Warning
  beta Prelookup : PreLookup  BreakpointsData=AeroCoeff.beta_prelookup  IndexSearchMethod=Linear search  BeginIndexSearchUsingPreviousIndexResult=on  DiagnosticForOutOfRangeInput=Warning
  dCn_beta : Interpolation_n-D  NumberOfTableDimensions=1  Table=AeroCoeff.dCn_beta
      settings: InputPortMap=u0,u1
  dCn_p_lef : Interpolation_n-D  NumberOfTableDimensions=1  Table=AeroCoeff.dCn_p_lef
      settings: InputPortMap=u0,u1
  dCn_r_lef : Interpolation_n-D  NumberOfTableDimensions=1  Table=AeroCoeff.dCn_r_lef
      settings: InputPortMap=u0,u1
  elevator Prelookup : PreLookup  BreakpointsData=AeroCoeff.elevator_prelookup1  IndexSearchMethod=Linear search  BeginIndexSearchUsingPreviousIndexResult=on  DiagnosticForOutOfRangeInput=Warning
  Cn_tot : Outport  VectorParamsAs1DForOutWhenUnconnected=off
  wires:
  alpha Prelookup/1 -> Cn/1, dCn_p_lef/1, dCn_beta/1, Cn_p/1, dCn_r_lef/1, Cn_r/1, Cn_delta_r/1, Cn_delta_ail_lef/1, Cn_delta_ail/1, Cn_elevator0/1, Cn_lef/1
  Add1/1 -> Add5/1, [delta_Cn_delta_ail], Add2/2
  Cn_elevator0/1 -> Add3/2, Add1/2, Add/2
  alpha Prelookup/2 -> Cn/2, Cn_lef/2, dCn_p_lef/2, dCn_beta/2, Cn_p/2, dCn_r_lef/2, Cn_r/2, Cn_delta_r/2, Cn_delta_ail_lef/2, Cn_delta_ail/2, Cn_elevator0/2
  elevator Prelookup/1 -> Cn/5
  Add6/1 -> Product5/2
  beta Prelookup/2 -> Cn_delta_r/4, Cn_delta_ail_lef/4, Cn_delta_ail/4, Cn/4, Cn_lef/4, Cn_elevator0/4
  Cn_r/1 -> Add6/1
  Cn_delta_ail_lef/1 -> Add2/3
  pb_2v/1 -> Product7/1
  Add5/1 -> Product2/1
  Cn_lef/1 -> Add2/1, Add/1
  Add4/1 -> Cn_tot/1
  Add7/1 -> Product7/2
  beta (deg)/1 -> Angle Conversion/1, beta Prelookup/1
  rb_2v/1 -> Product5/1
  Product10/1 -> Add4/9
  Add/1 -> Product/1
  x_cg/1 -> Add8/2
  alpha (deg)/1 -> alpha Prelookup/1
  b/1 -> Divide/2
  dCn_r_lef/1 -> Product4/2
  drud/1 -> Product3/2
  dCn_beta/1 -> Product8/1
  Product4/1 -> Add6/2
  Divide/1 -> Product10/2
  Product3/1 -> Add4/5
  x_cg_ref/1 -> Add8/1
  Cn_p/1 -> Add7/1
  dCn_p_lef/1 -> Product6/1
  Product8/1 -> Add4/8
  elevator Prelookup/2 -> Cn/6
  Cn_delta_r/1 -> Add3/1
  Product6/1 -> Add7/2
  Cy_tot/1 -> Product10/3
  Product7/1 -> Add4/7
  Product5/1 -> Add4/6
  Add2/1 -> Product1/1
  beta Prelookup/1 -> Cn_delta_r/3, Cn_delta_ail_lef/3, Cn_delta_ail/3, Cn/3, Cn_lef/3, Cn_elevator0/3
  Product2/1 -> Add4/4
  Cn/1 -> Add4/2
  Cn_delta_ail/1 -> Add1/1
  Add3/1 -> Product3/1
  dlef/1 -> Product6/2, Product4/1, Product/2, Product1/2
  Product/1 -> Add4/3
  Product1/1 -> Add5/2
  cbar/1 -> Divide/1
  Add8/1 -> Product10/1
  right aileron/1 -> Add9/1
  left aileron/1 -> Add9/2
  Add9/1 -> Gain/1
  Gain/1 -> Product2/2
  Add10/1 -> Gain4/1
  [delta_Cn_delta_ail] -> Gain2/1
  Gain1/1 -> Product9/2
  Gain2/1 -> Product9/1
  Product9/1 -> Add4/1
  "right elevator (deg) "/1 -> Add11/1, Add10/1
  left elevator (deg)/1 -> Add11/2, Add10/2
  Add11/1 -> Gain1/1
  Gain4/1 -> elevator Prelookup/1
  Angle Conversion/1 -> Product8/2

== system Copy_of_NDI/F-16 Vehicle Systems Model/Vehicle/Aerodynamics/Aerofynamic Coefficients/Ground Effects ==
  alpha (deg) : Inport
  beta(deg) : Inport  Port=2
  h_AGL : Inport  Port=3
  Coeff : Outport

== system Copy_of_NDI/F-16 Vehicle Systems Model/Vehicle/Aerodynamics/Aerofynamic Coefficients/Landing Gear Effects ==
  alpha (deg) : Inport
  beta(deg) : Inport  Port=2
  Landing Gear Angle : Inport  Port=3
  Coeff : Outport

== system Copy_of_NDI/F-16 Vehicle Systems Model/Vehicle/LandingGear GroundReaction/L Main Gear Geometry Forces and Moments/Calc Gear Force and Pos ==
  note: 註:令[ XcB YcB ZcB ] = [ 0 0 0 ]
  note: 詹庭宇:此Block正負號為+---
  note: $∆z_g^B$
  note: $∆z_g^b =z_g^b -z_g^{b^{\prime } } =z_g^b -\frac{z_r^E -z_c^E -C_{31} {\left(x_g^b -x_c^b \right)}-C_{32} {\left(y_g^b -y_c^b \right)}}{C_{33} }$
  note: $z_r^E =z_c^E +C_{31} {\left(x_g^b -x_c^b \right)}+C_{32} {\left(y_g^b -y_c^b \right)}+C_{33} \cdot z_g^{b^{\prime } }$
  note: $z_g^E =z_c^E +C_{31} {\left(x_g^b -x_c^b \right)}+C_{32} {\left(y_g^b -y_c^b \right)}+C_{33} {\left(z_g^b -z_c^b \right)}$
  note: $p^E ={\left[C\right]}{\left(p^b -p_c^b \right)}+p_c^E$
  note: $\left(p^E -p_c^E \right)={\left[C\right]}{\left(p^b -p_c^b \right)}$
  note: 定義：
      | 慣性座標+Z軸朝下
      | 體座標+Z軸朝下
  WOW : Inport
  ZrL : Inport  Port=2
  Xg : Inport  Port=3
  ZcL : Inport  Port=4
  DCM_eb : Inport  Port=5
  Constant : Constant  Value=0
  Demux1 : Demux  Outputs=3
  Demux2 : Demux  Outputs=3
  RangeLimit : Saturate  UpperLimit=LandingGear.LM.CmprsRangeLimitUpper  LowerLimit=LandingGear.LM.CmprsRangeLimitLower
  Subsystem : Subsystem
  Sum1 : Sum  Inputs=+---
  Sum2 : Sum  Inputs=+-
  Switch : Switch  Criteria=u2 ~= 0  Threshold=243  SaturateOnIntegerOverflow=off  InputSameDT=off
  compression : Product  Inputs=*/  RndMeth=Zero
  get_row3 : Selector  NumberOfDimensions=2  InputPortWidth=3  IndexOptions=Index vector (dialog),Select all  Indices=3,-1  OutputSizes=1
  prod1 : Product  RndMeth=Zero
  prod2 : Product  RndMeth=Zero
  dZ_strut : Outport
  Fn_strut : Outport  Port=2
  ZgB_prime : Outport  Port=3
  wires:
  ZrL/1 -> Sum1/1
  DCM_eb/1 -> get_row3/1
  get_row3/1 -> Demux1/1  "C3"
  Demux1/1 -> prod1/2  "C31"
  Demux1/2 -> prod2/2  "C32"
  Demux2/1 -> prod1/1  "XgB-XcB"
  Demux2/2 -> prod2/1  "YgB-YcB"
  prod1/1 -> Sum1/3
  prod2/1 -> Sum1/4
  Demux1/3 -> compression/2, Subsystem/2(C33)  "C33"
  Subsystem/2(Fn_strut) -> Fn_strut/1
  compression/1 -> Sum2/2, ZgB_prime/1
  ZcL/1 -> Sum1/2
  Xg/1 -> Demux2/1
  Sum1/1 -> compression/1  "Strut_dZnum"
  Demux2/3 -> Sum2/1  "ZgB-ZcB"
  Subsystem/1(dZ_strut) -> dZ_strut/1
  RangeLimit/1 -> Subsystem/1(deltaZgB)
  Switch/1 -> RangeLimit/1
  Sum2/1 -> Switch/1  "T command"
  WOW/1 -> Switch/2
  Constant/1 -> Switch/3  "T command"

== system Copy_of_NDI/F-16 Vehicle Systems Model/Vehicle/LandingGear GroundReaction/L Main Gear Geometry Forces and Moments/GenerateGroundFM ==
  note: 正負號可能相反
  note: 慣性座標轉至體座標的旋轉矩陣
  note: 詹庭宇:拿掉/忽略輪胎側向力模型，Fy=0
  note: 詹庭宇:拿掉/忽略輪胎側向力模型，Fy=0
  GearLoc : Inport
  Fn_strut : Inport  Port=2
  ZgB_prime : Inport  Port=3
  DCM_be : Inport  Port=4
  plant : Inport  Port=5
  Enable : EnablePort
  Constant : Constant  Value=0
  Constant1 : Constant  Value=[0 0 0]
  Demux : Demux  Outputs=3
  Forces and distances to LMN : Subsystem
  Gear Local Force vector : Concatenate  NumInputs=3  Mode=Multidimensional array
  LocMatrix1 : Subsystem
  Local Forces to Body Axes : Product  Multiplication=Matrix(*)  InputSameDT=on  SaturateOnIntegerOverflow=on  OutDataTypeStr=Inherit: Same as first input
  Manual Switch : ManualSwitch  CurrentSetting=0
  Moments about CG due to Forces : aerolibbdyn/Moments about CG  due to Forces
  Mux1 : Mux  Inputs=2
  Mux2 : Mux  Inputs=3
  Rotation Speed(TVC ON) : Subsystem
  Terminator : Terminator
  FM : Outport
  wires:
  DCM_be/1 -> Local Forces to Body Axes/1
  Mux1/1 -> FM/1
  Local Forces to Body Axes/1 -> Moments about CG due to Forces/1, Forces and distances to LMN/1(Fb)
  Gear Local Force vector/1 -> Local Forces to Body Axes/2, Mux1/1
  Constant/1 -> Gear Local Force vector/2
  ZgB_prime/1 -> Mux2/3, LocMatrix1/2(ZgB_prime)
  Forces and distances to LMN/1(LMNe) -> Manual Switch/1
  Manual Switch/1 -> Mux1/2
  Moments about CG due to Forces/1 -> Manual Switch/2
  Constant1/1 -> Moments about CG due to Forces/2
  LocMatrix1/1(A) -> Forces and distances to LMN/2(Xg_gnd)
  Demux/1 -> Mux2/1
  Demux/3 -> Terminator/1
  GearLoc/1 -> Demux/1, LocMatrix1/1(XgB)
  Mux2/1 -> Moments about CG due to Forces/3
  Demux/2 -> Mux2/2
  plant/1 -> Rotation Speed(TVC ON)/2(PlantData)
  Fn_strut/1 -> Gear Local Force vector/3, Rotation Speed(TVC ON)/1(friction)
  Rotation Speed(TVC ON)/1(output) -> Gear Local Force vector/1

== system Copy_of_NDI/F-16 Vehicle Systems Model/Vehicle/LandingGear GroundReaction/Nose Gear Geometry Forces and Moments/Calc Gear Force and Pos ==
  note: 註:令[ XcB YcB ZcB ] = [ 0 0 0 ]
  note: 詹庭宇:此Block正負號為+---
  note: $∆z_g^B$
  note: $∆z_g^b =z_g^b -z_g^{b^{\prime } } =z_g^b -\frac{z_r^E -z_c^E -C_{31} {\left(x_g^b -x_c^b \right)}-C_{32} {\left(y_g^b -y_c^b \right)}}{C_{33} }$
  note: $z_r^E =z_c^E +C_{31} {\left(x_g^b -x_c^b \right)}+C_{32} {\left(y_g^b -y_c^b \right)}+C_{33} \cdot z_g^{b^{\prime } }$
  note: $z_g^E =z_c^E +C_{31} {\left(x_g^b -x_c^b \right)}+C_{32} {\left(y_g^b -y_c^b \right)}+C_{33} {\left(z_g^b -z_c^b \right)}$
  note: $p^E ={\left[C\right]}{\left(p^b -p_c^b \right)}+p_c^E$
  note: $\left(p^E -p_c^E \right)={\left[C\right]}{\left(p^b -p_c^b \right)}$
  note: 定義：
      | 慣性座標+Z軸朝下
      | 體座標+Z軸朝下
  WOW : Inport
  ZrL : Inport  Port=2
  Xg : Inport  Port=3
  ZcL : Inport  Port=4
  DCM_eb : Inport  Port=5
  Constant : Constant  Value=0
  Demux1 : Demux  Outputs=3
  Demux2 : Demux  Outputs=3
  RangeLimit : Saturate  UpperLimit=LandingGear.Nose.CmprsRangeLimitUpper  LowerLimit=LandingGear.Nose.CmprsRangeLimitLower
  Subsystem : Subsystem
  Sum1 : Sum  Inputs=+---
  Sum2 : Sum  Inputs=+-
  Switch : Switch  Criteria=u2 ~= 0  Threshold=243  SaturateOnIntegerOverflow=off  InputSameDT=off
  compression : Product  Inputs=*/  RndMeth=Zero
  get_row3 : Selector  NumberOfDimensions=2  InputPortWidth=3  IndexOptions=Index vector (dialog),Select all  Indices=3,-1  OutputSizes=1
  prod1 : Product  RndMeth=Zero
  prod2 : Product  RndMeth=Zero
  dZ_strut : Outport
  Fn_strut : Outport  Port=2
  ZgB_prime : Outport  Port=3
  wires:
  ZrL/1 -> Sum1/1
  DCM_eb/1 -> get_row3/1
  get_row3/1 -> Demux1/1  "C3"
  Demux1/1 -> prod1/2  "C31"
  Demux1/2 -> prod2/2  "C32"
  Demux2/1 -> prod1/1  "XgB-XcB"
  Demux2/2 -> prod2/1  "YgB-YcB"
  prod1/1 -> Sum1/3
  prod2/1 -> Sum1/4
  Demux1/3 -> compression/2, Subsystem/2(C33)  "C33"
  Subsystem/2(Fn_strut) -> Fn_strut/1
  compression/1 -> Sum2/2, ZgB_prime/1
  ZcL/1 -> Sum1/2
  Xg/1 -> Demux2/1
  Sum1/1 -> compression/1  "Strut_dZnum"
  Demux2/3 -> Sum2/1  "ZgB-ZcB"
  Subsystem/1(dZ_strut) -> dZ_strut/1
  RangeLimit/1 -> Subsystem/1(deltaZgB)
  Switch/1 -> RangeLimit/1
  Sum2/1 -> Switch/1  "T command"
  WOW/1 -> Switch/2
  Constant/1 -> Switch/3  "T command"

== system Copy_of_NDI/F-16 Vehicle Systems Model/Vehicle/LandingGear GroundReaction/Nose Gear Geometry Forces and Moments/GenerateGroundFM ==
  note: 正負號可能相反
  note: 慣性座標轉至體座標的旋轉矩陣
  note: 詹庭宇:拿掉/忽略輪胎側向力模型，Fy=0
  note: 詹庭宇:拿掉/忽略輪胎側向力模型，Fy=0
  GearLoc : Inport
  Fn_strut : Inport  Port=2
  ZgB_prime : Inport  Port=3
  DCM_be : Inport  Port=4
  plant : Inport  Port=5
  Enable : EnablePort
  Constant : Constant  Value=0
  Constant1 : Constant  Value=[0 0 0]
  Demux : Demux  Outputs=3
  Forces and distances to LMN : Subsystem
  Gear Local Force vector : Concatenate  NumInputs=3  Mode=Multidimensional array
  LocMatrix1 : Subsystem
  Local Forces to Body Axes : Product  Multiplication=Matrix(*)  InputSameDT=on  SaturateOnIntegerOverflow=on  OutDataTypeStr=Inherit: Same as first input
  Manual Switch : ManualSwitch  CurrentSetting=0
  Moments about CG due to Forces : aerolibbdyn/Moments about CG  due to Forces
  Mux1 : Mux  Inputs=2
  Mux2 : Mux  Inputs=3
  Rotation Speed(TVC ON) : Subsystem
  Terminator : Terminator
  FM : Outport
  wires:
  DCM_be/1 -> Local Forces to Body Axes/1
  Mux1/1 -> FM/1
  Local Forces to Body Axes/1 -> Moments about CG due to Forces/1, Forces and distances to LMN/1(Fb)
  Gear Local Force vector/1 -> Local Forces to Body Axes/2, Mux1/1
  Constant/1 -> Gear Local Force vector/2
  ZgB_prime/1 -> Mux2/3, LocMatrix1/2(ZgB_prime)
  Forces and distances to LMN/1(LMNe) -> Manual Switch/1
  Manual Switch/1 -> Mux1/2
  Moments about CG due to Forces/1 -> Manual Switch/2
  Constant1/1 -> Moments about CG due to Forces/2
  LocMatrix1/1(A) -> Forces and distances to LMN/2(Xg_gnd)
  Demux/1 -> Mux2/1
  Demux/3 -> Terminator/1
  GearLoc/1 -> Demux/1, LocMatrix1/1(XgB)
  Mux2/1 -> Moments about CG due to Forces/3
  Demux/2 -> Mux2/2
  plant/1 -> Rotation Speed(TVC ON)/2(PlantData)
  Fn_strut/1 -> Gear Local Force vector/3, Rotation Speed(TVC ON)/1(friction)
  Rotation Speed(TVC ON)/1(output) -> Gear Local Force vector/1

== system Copy_of_NDI/F-16 Vehicle Systems Model/Vehicle/LandingGear GroundReaction/R Main Gear Geometry Forces and Moments/Calc Gear Force and Pos ==
  note: 註:令[ XcB YcB ZcB ] = [ 0 0 0 ]
  note: 詹庭宇:此Block正負號為+---
  note: $∆z_g^B$
  note: $∆z_g^b =z_g^b -z_g^{b^{\prime } } =z_g^b -\frac{z_r^E -z_c^E -C_{31} {\left(x_g^b -x_c^b \right)}-C_{32} {\left(y_g^b -y_c^b \right)}}{C_{33} }$
  note: $z_r^E =z_c^E +C_{31} {\left(x_g^b -x_c^b \right)}+C_{32} {\left(y_g^b -y_c^b \right)}+C_{33} \cdot z_g^{b^{\prime } }$
  note: $z_g^E =z_c^E +C_{31} {\left(x_g^b -x_c^b \right)}+C_{32} {\left(y_g^b -y_c^b \right)}+C_{33} {\left(z_g^b -z_c^b \right)}$
  note: $p^E ={\left[C\right]}{\left(p^b -p_c^b \right)}+p_c^E$
  note: $\left(p^E -p_c^E \right)={\left[C\right]}{\left(p^b -p_c^b \right)}$
  note: 定義：
      | 慣性座標+Z軸朝下
      | 體座標+Z軸朝下
  WOW : Inport
  ZrL : Inport  Port=2
  Xg : Inport  Port=3
  ZcL : Inport  Port=4
  DCM_eb : Inport  Port=5
  Constant : Constant  Value=0
  Demux1 : Demux  Outputs=3
  Demux2 : Demux  Outputs=3
  RangeLimit : Saturate  UpperLimit=LandingGear.RM.CmprsRangeLimitUpper  LowerLimit=LandingGear.RM.CmprsRangeLimitLower
  Subsystem : Subsystem
  Sum1 : Sum  Inputs=+---
  Sum2 : Sum  Inputs=+-
  Switch : Switch  Criteria=u2 ~= 0  Threshold=243  SaturateOnIntegerOverflow=off  InputSameDT=off
  compression : Product  Inputs=*/  RndMeth=Zero
  get_row3 : Selector  NumberOfDimensions=2  InputPortWidth=3  IndexOptions=Index vector (dialog),Select all  Indices=3,-1  OutputSizes=1
  prod1 : Product  RndMeth=Zero
  prod2 : Product  RndMeth=Zero
  dZ_strut : Outport
  Fn_strut : Outport  Port=2
  ZgB_prime : Outport  Port=3
  wires:
  ZrL/1 -> Sum1/1
  DCM_eb/1 -> get_row3/1
  get_row3/1 -> Demux1/1  "C3"
  Demux1/1 -> prod1/2  "C31"
  Demux1/2 -> prod2/2  "C32"
  Demux2/1 -> prod1/1  "XgB-XcB"
  Demux2/2 -> prod2/1  "YgB-YcB"
  prod1/1 -> Sum1/3
  prod2/1 -> Sum1/4
  Demux1/3 -> compression/2, Subsystem/2(C33)  "C33"
  Subsystem/2(Fn_strut) -> Fn_strut/1
  compression/1 -> Sum2/2, ZgB_prime/1
  ZcL/1 -> Sum1/2
  Xg/1 -> Demux2/1
  Sum1/1 -> compression/1  "Strut_dZnum"
  Demux2/3 -> Sum2/1  "ZgB-ZcB"
  Subsystem/1(dZ_strut) -> dZ_strut/1
  RangeLimit/1 -> Subsystem/1(deltaZgB)
  Switch/1 -> RangeLimit/1
  Sum2/1 -> Switch/1  "T command"
  WOW/1 -> Switch/2
  Constant/1 -> Switch/3  "T command"

== system Copy_of_NDI/F-16 Vehicle Systems Model/Vehicle/LandingGear GroundReaction/R Main Gear Geometry Forces and Moments/GenerateGroundFM ==
  note: 正負號可能相反
  note: 慣性座標轉至體座標的旋轉矩陣
  note: 詹庭宇:拿掉/忽略輪胎側向力模型，Fy=0
  note: 詹庭宇:拿掉/忽略輪胎側向力模型，Fy=0
  GearLoc : Inport
  Fn_strut : Inport  Port=2
  ZgB_prime : Inport  Port=3
  DCM_be : Inport  Port=4
  plant : Inport  Port=5
  Enable : EnablePort
  Constant : Constant  Value=0
  Constant1 : Constant  Value=[0 0 0]
  Demux : Demux  Outputs=3
  Forces and distances to LMN : Subsystem
  Gear Local Force vector : Concatenate  NumInputs=3  Mode=Multidimensional array
  LocMatrix1 : Subsystem
  Local Forces to Body Axes : Product  Multiplication=Matrix(*)  InputSameDT=on  SaturateOnIntegerOverflow=on  OutDataTypeStr=Inherit: Same as first input
  Manual Switch : ManualSwitch  CurrentSetting=0
  Moments about CG due to Forces : aerolibbdyn/Moments about CG  due to Forces
  Mux1 : Mux  Inputs=2
  Mux2 : Mux  Inputs=3
  Rotation Speed(TVC ON) : Subsystem
  Terminator : Terminator
  FM : Outport
  wires:
  DCM_be/1 -> Local Forces to Body Axes/1
  Mux1/1 -> FM/1
  Local Forces to Body Axes/1 -> Moments about CG due to Forces/1, Forces and distances to LMN/1(Fb)
  Gear Local Force vector/1 -> Local Forces to Body Axes/2, Mux1/1
  Constant/1 -> Gear Local Force vector/2
  ZgB_prime/1 -> Mux2/3, LocMatrix1/2(ZgB_prime)
  Forces and distances to LMN/1(LMNe) -> Manual Switch/1
  Manual Switch/1 -> Mux1/2
  Moments about CG due to Forces/1 -> Manual Switch/2
  Constant1/1 -> Moments about CG due to Forces/2
  LocMatrix1/1(A) -> Forces and distances to LMN/2(Xg_gnd)
  Demux/1 -> Mux2/1
  Demux/3 -> Terminator/1
  GearLoc/1 -> Demux/1, LocMatrix1/1(XgB)
  Mux2/1 -> Moments about CG due to Forces/3
  Demux/2 -> Mux2/2
  plant/1 -> Rotation Speed(TVC ON)/2(PlantData)
  Fn_strut/1 -> Gear Local Force vector/3, Rotation Speed(TVC ON)/1(friction)
  Rotation Speed(TVC ON)/1(output) -> Gear Local Force vector/1

== system Copy_of_NDI/F-16 Vehicle Systems Model/Vehicle/Propulsion/Afterburning Turbofan Jet Engine/If Action Subsystem ==
  note: Pow_max
      |
      | Pow_min
      |
      | T_idle
      |
      | T_mil
      |
      | T_max
  "input " : Inport
  Action Port : ActionPort
  Add : Sum
  Add1 : Sum  Inputs=-+
  Demux : Demux  Outputs=5
  Divide : Product  Inputs=**
  Gain : Gain  Gain=1/50
  Terminator : Terminator
  Terminator1 : Terminator
  T_max1 : Outport  VectorParamsAs1DForOutWhenUnconnected=off
  wires:
  Demux/3 -> Add1/1, Add/1
  Demux/4 -> Add1/2
  Add1/1 -> Divide/2
  Gain/1 -> Divide/1
  Divide/1 -> Add/2
  Add/1 -> T_max1/1
  "input "/1 -> Demux/1
  Demux/1 -> Gain/1
  Demux/2 -> Terminator/1
  Demux/5 -> Terminator1/1

== system Copy_of_NDI/F-16 Vehicle Systems Model/Vehicle/Propulsion/Afterburning Turbofan Jet Engine/If Action Subsystem1 ==
  note: Pow_max
      |
      | Pow_min
      |
      | T_idle
      |
      | T_mil
      |
      | T_max
  "input " : Inport
  Action Port : ActionPort
  Add : Sum
  Add1 : Sum  Inputs=-+
  Add2 : Sum  Inputs=-+
  Constant : Constant  Value=50
  Demux : Demux  Outputs=5
  Gain : Gain  Gain=1/50
  Product : Product
  Terminator : Terminator
  Terminator1 : Terminator
  T_max1 : Outport  VectorParamsAs1DForOutWhenUnconnected=off
  wires:
  "input "/1 -> Demux/1
  Demux/4 -> Add/2, Add1/1
  Demux/5 -> Add1/2
  Demux/1 -> Add2/2
  Constant/1 -> Add2/1
  Add2/1 -> Gain/1
  Add1/1 -> Product/2
  Gain/1 -> Product/1
  Product/1 -> Add/1
  Add/1 -> T_max1/1
  Demux/3 -> Terminator1/1
  Demux/2 -> Terminator/1

== system Copy_of_NDI/F-16 Vehicle Systems Model/Vehicle/Propulsion/Afterburning Turbofan Jet Engine/If Action Subsystem2 ==
  note: Pow_max
      |
      | Pow_min
      |
      | T_idle
      |
      | T_mil
      |
      | T_max
  "input " : Inport
  Action Port : ActionPort
  Add : Sum
  Add1 : Sum  Inputs=-+
  Demux : Demux  Outputs=5
  Divide : Product  Inputs=**
  Gain : Gain  Gain=1/50
  Terminator : Terminator
  Terminator1 : Terminator
  T_min : Outport  VectorParamsAs1DForOutWhenUnconnected=off
  wires:
  Demux/3 -> Add1/1, Add/1
  Demux/4 -> Add1/2
  Add1/1 -> Divide/2
  Gain/1 -> Divide/1
  Divide/1 -> Add/2
  Add/1 -> T_min/1
  "input "/1 -> Demux/1
  Demux/2 -> Gain/1
  Demux/5 -> Terminator1/1
  Demux/1 -> Terminator/1

== system Copy_of_NDI/F-16 Vehicle Systems Model/Vehicle/Propulsion/Afterburning Turbofan Jet Engine/If Action Subsystem3 ==
  note: Pow_max
      |
      | Pow_min
      |
      | T_idle
      |
      | T_mil
      |
      | T_max
  "input " : Inport
  Action Port : ActionPort
  Add : Sum
  Add1 : Sum  Inputs=-+
  Add2 : Sum  Inputs=-+
  Constant : Constant  Value=50
  Demux : Demux  Outputs=5
  Gain : Gain  Gain=1/50
  Product : Product
  Terminator : Terminator
  Terminator1 : Terminator
  T_min : Outport  VectorParamsAs1DForOutWhenUnconnected=off
  wires:
  "input "/1 -> Demux/1
  Demux/4 -> Add/2, Add1/1
  Demux/5 -> Add1/2
  Constant/1 -> Add2/1
  Add2/1 -> Gain/1
  Add1/1 -> Product/2
  Gain/1 -> Product/1
  Product/1 -> Add/1
  Add/1 -> T_min/1
  Demux/3 -> Terminator1/1
  Demux/2 -> Add2/2
  Demux/1 -> Terminator/1

== system Copy_of_NDI/F-16 Vehicle Systems Model/Vehicle/Propulsion/Afterburning Turbofan Jet Engine/If Action Subsystem4 ==
  In1 : Inport
  Action Port : ActionPort
  Out1 : Outport
  wires:
  In1/1 -> Out1/1

== system Copy_of_NDI/F-16 Vehicle Systems Model/Vehicle/Propulsion/Afterburning Turbofan Jet Engine/If Action Subsystem5 ==
  In1 : Inport
  Action Port : ActionPort
  Out1 : Outport
  wires:
  In1/1 -> Out1/1

== system Copy_of_NDI/F-16 Vehicle Systems Model/Vehicle/Propulsion/Afterburning Turbofan Jet Engine/If Action Subsystem6 ==
  In1 : Inport
  Action Port : ActionPort
  Out1 : Outport
  wires:
  In1/1 -> Out1/1

== system Copy_of_NDI/F-16 Vehicle Systems Model/Vehicle/Propulsion(two_nozzles)/Afterburning Turbofan Jet Engine/If Action Subsystem ==
  note: Pow_max
      |
      | Pow_min
      |
      | T_idle
      |
      | T_mil
      |
      | T_max
  "input " : Inport
  Action Port : ActionPort  ActionPortLabel=if(u1<50)
  Add : Sum
  Add1 : Sum  Inputs=-+
  Demux : Demux  Outputs=5
  Divide : Product  Inputs=**
  Gain : Gain  Gain=1/50
  Terminator : Terminator
  Terminator1 : Terminator
  T_max1 : Outport  VectorParamsAs1DForOutWhenUnconnected=off
  wires:
  Demux/3 -> Add1/1, Add/1
  Demux/4 -> Add1/2
  Add1/1 -> Divide/2
  Gain/1 -> Divide/1
  Divide/1 -> Add/2
  Add/1 -> T_max1/1
  "input "/1 -> Demux/1
  Demux/1 -> Gain/1
  Demux/2 -> Terminator/1
  Demux/5 -> Terminator1/1

== system Copy_of_NDI/F-16 Vehicle Systems Model/Vehicle/Propulsion(two_nozzles)/Afterburning Turbofan Jet Engine/If Action Subsystem1 ==
  note: Pow_max
      |
      | Pow_min
      |
      | T_idle
      |
      | T_mil
      |
      | T_max
  "input " : Inport
  Action Port : ActionPort  ActionPortLabel=elseif(u1>=50)
  Add : Sum
  Add1 : Sum  Inputs=-+
  Add2 : Sum  Inputs=-+
  Constant : Constant  Value=50
  Demux : Demux  Outputs=5
  Gain : Gain  Gain=1/50
  Product : Product
  Terminator : Terminator
  Terminator1 : Terminator
  T_max1 : Outport  VectorParamsAs1DForOutWhenUnconnected=off
  wires:
  "input "/1 -> Demux/1
  Demux/4 -> Add/2, Add1/1
  Demux/5 -> Add1/2
  Demux/1 -> Add2/2
  Constant/1 -> Add2/1
  Add2/1 -> Gain/1
  Add1/1 -> Product/2
  Gain/1 -> Product/1
  Product/1 -> Add/1
  Add/1 -> T_max1/1
  Demux/3 -> Terminator1/1
  Demux/2 -> Terminator/1
